simulink model "Separately_excited_DC_motor"  (R2024a)
settings: Solver=ode15s  StartTime=0.0  StopTime=35  RelTol=1e-3
values from neighbouring files (symbols this model uses):
  A = 1.4    [CruiseControl.m]
libraries: slpidlib x2, spsControlledVoltageSourceLib x2, spsGroundLib x2, spsDCMachineLib x1, SignalEditorBlockLib x1, sps_lib x1
settings Model: Creator=macbookair  LastModifiedBy=macbookair

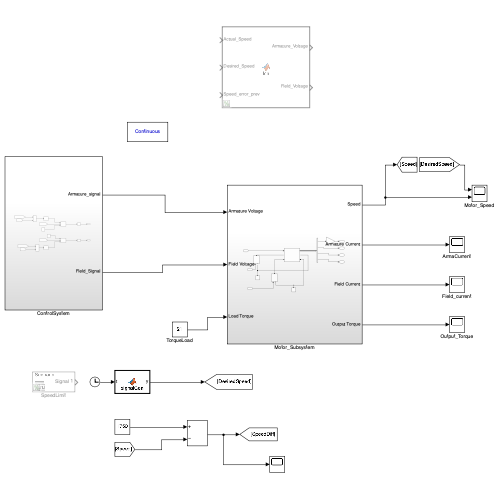
[thumbnail: Simulink's stored preview of the top-level diagram]
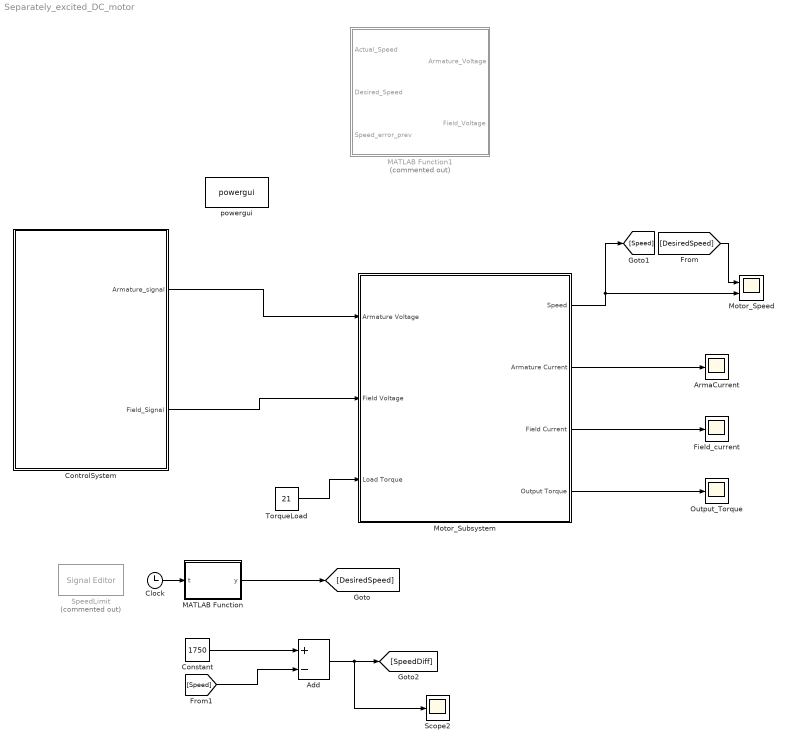
== system Separately_excited_DC_motor ==
  Add : Sum  Inputs=+-
  ArmaCurrent : Scope
  Clock : Clock
  Constant : Constant  Value=1750
  ControlSystem : Subsystem
  Field_current : Scope
  MATLAB Function : MATLAB Function  TreatAsAtomicUnit=on
  MATLAB Function1 : MATLAB Function  Commented=on  TreatAsAtomicUnit=on
  Motor_Speed : Scope  NumInputPorts=2
  Motor_Subsystem : Subsystem
  Output_Torque : Scope
  Scope2 : Scope
  SpeedLimit : SignalEditorBlockLib/Signal Editor  Commented=on  FileName=SpeedLimit.mat  ActiveScenario=Scenario  ActiveSignal=Signal 1  IsBus=off  OutputBusObjectStr=Bus: BusObject  SampleTime=0  Interpolate=off  ZeroCross=off  OutputAfterFinalValue=Setting to zero  Unit=inherit  PreserveSignalName=on  ApplySigPropsToAllScenarios=on  ApplySigPropsToAllSignals=off
  TorqueLoad : Constant  Value=21
  powergui : sps_lib/powergui  Priority=1  SimulationMode=Continuous  SampleTime=50e-6  frequency=60  Iterations=50  frequencyindice=0  Pbase=100e6  ErrMax=1e-4  UnitsV=kV  UnitsW=MW  buscounter=0  FunctionMessages=off  echomessages=off  EnableUseOfTLC=off  CurrentSourceSwitches=off  DisableSnubberDevices=off  DisableRonSwitches=off  DisableVfSwitches=off  DisplayEquations=off  AutomaticDiscreteSolvers=off  SolverType=Tustin/Backward Euler (TBE)  Interpol=off  ExternalGateDelay=off  methode=off  Ts=100  x0status=blocks  SPID=on  SwTol=0  HookPort=off  NonlinearTolerance=1e-4  nMaxIteration=100  ContinueOnMaxIteration=off  RestoreLinks=warning  ResistiveCurrentMeasurement=off  Frange=[0:2:500]  Ylog=off  Xlog=on  ShowGrid=off  save=off  variable=ZData  structure=0  ZoomFFT=off  StartTime=0.0  cycles=1  DisplayStyle=1  fundamental=60  FreqAxis=off  MaxFrequency=1000  frequencyindicesteady=1  RmsSteady=1  display=off
  wires:
  Motor_Subsystem/2(Armature Current) -> ArmaCurrent/1
  Motor_Subsystem/4(Output Torque) -> Output_Torque/1
  Motor_Subsystem/3(Field Current) -> Field_current/1
  Motor_Subsystem/1(Speed) -> Motor_Speed/2, [Speed]
  [DesiredSpeed] -> Motor_Speed/1
  [Speed] -> Add/2
  Constant/1 -> Add/1
  Add/1 -> Scope2/1, [SpeedDiff]
  TorqueLoad/1 -> Motor_Subsystem/3(Load Torque)
  Clock/1 -> MATLAB Function/1(t)
  MATLAB Function/1(y) -> [DesiredSpeed]
  ControlSystem/1(Armature_signal) -> Motor_Subsystem/1(Armature Voltage)
  ControlSystem/2(Field_Signal) -> Motor_Subsystem/2(Field Voltage)

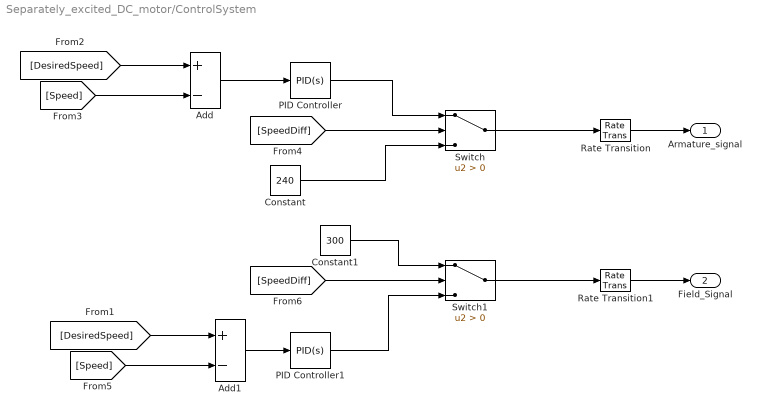
== system Separately_excited_DC_motor/ControlSystem ==
  Add : Sum  Inputs=+-
  Add1 : Sum  Inputs=+-
  Constant : Constant  Value=240
  Constant1 : Constant  Value=300
  PID Controller : slpidlib/PID Controller  Controller=PID  Form=Parallel  TimeDomain=Continuous-time  UseExternalTs=off  SampleTime=-1  IntegratorMethod=Forward Euler  FilterMethod=Forward Euler  ControllerParametersSource=internal  P=100  I=50  UseKiTs=off  D=0.001  UseExternalDerivativeSource=off  N=100  UseFilter=on  TunerSelectOption=Transfer Function Based (PID Tuner App)  InitialConditionSource=internal  InitialConditionForIntegrator=0  InitialConditionForFilter=0  DifferentiatorICPrevScaledInput=0  ExternalReset=none  TrackingMode=off  Kt=1  LimitOutput=off  SatLimitsSource=internal  UpperSaturationLimit=inf  LowerSaturationLimit=-inf  LinearizeAsGain=on  AntiWindupMode=none  Kb=1  LimitIntegrator=off  UpperIntegratorSaturationLimit=inf  LowerIntegratorSaturationLimit=-inf  POutMin=[]  POutMax=[]  IOutMin=[]  IOutMax=[]  DOutMin=[]  DOutMax=[]  NOutMin=[]  NOutMax=[]  SumOutMin=[]  SumOutMax=[]  SaturationOutMin=[]  SaturationOutMax=[]  PParamMin=[]  PParamMax=[]  IParamMin=[]  IParamMax=[]  DParamMin=[]  DParamMax=[]  NParamMin=[]  NParamMax=[]  KbParamMin=[]  KbParamMax=[]  KtParamMin=[]  KtParamMax=[]  KbOutMin=[]  KbOutMax=[]  KtOutMin=[]  KtOutMax=[]  IntegratorOutMin=[]  IntegratorOutMax=[]  FilterOutMin=[]  FilterOutMax=[]  SumI1OutMin=[]  SumI1OutMax=[]  SumI2OutMin=[]  SumI2OutMax=[]  SumI3OutMin=[]  SumI3OutMax=[]  SumI4OutMin=[]  SumI4OutMax=[]  SumDOutMin=[]  SumDOutMax=[]  DifferentiatorOutMin=[]  DifferentiatorOutMax=[]  FilterDiffOutCoefMin=[]  FilterDiffOutCoefMax=[]  ReciprocalOutMin=[]  ReciprocalOutMax=[]  SumDenOutMin=[]  SumDenOutMax=[]  SumNumOutMin=[]  SumNumOutMax=[]  DivideOutMin=[]  DivideOutMax=[]  UdiffTsProdOutMin=[]  UdiffTsProdOutMax=[]  NTsProdOutMin=[]  NTsProdOutMax=[]  UintegralTsProdOutMin=[]  UintegralTsProdOutMax=[]  UngainTsProdOutMin=[]  UngainTsProdOutMax=[]  ClampingZeroOutDataTypeStr=Inherit: Inherit via back propagation  ClampingZeroOutMin=[]  ClampingZeroOutMax=[]  FilterDenConstantOutDataTypeStr=Inherit: Inherit via back propagation  FilterDenConstantOutMin=[]  FilterDenConstantOutMax=[]  PCopyOutDataTypeStr=Inherit: Inherit via back propagation  PCopyOutMin=[]  PCopyOutMax=[]  NCopyOutDataTypeStr=Inherit: Inherit via back propagation  NCopyOutMin=[]  NCopyOutMax=[]  IntegratorContinuousStateAttributes=''  IntegratorStateMustResolveToSignalObject=off  IntegratorRTWStateStorageClass=Auto  FilterContinuousStateAttributes=''  FilterStateMustResolveToSignalObject=off  FilterRTWStateStorageClass=Auto  ParallelPVariant=InternalParameters  IdealPVariant=Disabled  IVariant=InternalParameters  DVariant=InternalParameters  IntegratorVariant=Continuous  SatVariant=Disabled  AWVariant=Passthrough  PCopyVariant=Disabled  TRVariant=Disabled  FdbkBlocksVariant=Forward  IdealPFdbkVariant=Disabled  SatFdbkVariant=Disabled  DerivativeFilterVariant=ContFilter  NVariant=InternalParameters  NCopyVariant=Disabled  FilterICVariant=InternalICsFilter  IntegratorICVariant=InternalICs  ExternalResetVariant=Disabled  TRSumVariant=Passthrough  SumFdbkVariant=Disabled  SumVariant=Sum_PID  TsampFilterVariant=InternalTs  TsampNgainVariant=Passthrough  TsampIntegralVariant=Disabled_SignalSpec  ExternalSaturationOutDataTypeStr=Inherit: Same as second input  DerivativeSourceVariant=ErrorSignal
  PID Controller1 : slpidlib/PID Controller  Controller=PID  Form=Parallel  TimeDomain=Continuous-time  UseExternalTs=off  SampleTime=-1  IntegratorMethod=Forward Euler  FilterMethod=Forward Euler  ControllerParametersSource=internal  P=200  I=40  UseKiTs=off  D=0.001  UseExternalDerivativeSource=off  N=100  UseFilter=on  TunerSelectOption=Transfer Function Based (PID Tuner App)  InitialConditionSource=internal  InitialConditionForIntegrator=0  InitialConditionForFilter=0  DifferentiatorICPrevScaledInput=0  ExternalReset=none  TrackingMode=off  Kt=1  LimitOutput=off  SatLimitsSource=internal  UpperSaturationLimit=inf  LowerSaturationLimit=-inf  LinearizeAsGain=on  AntiWindupMode=none  Kb=1  LimitIntegrator=off  UpperIntegratorSaturationLimit=inf  LowerIntegratorSaturationLimit=-inf  POutMin=[]  POutMax=[]  IOutMin=[]  IOutMax=[]  DOutMin=[]  DOutMax=[]  NOutMin=[]  NOutMax=[]  SumOutMin=[]  SumOutMax=[]  SaturationOutMin=[]  SaturationOutMax=[]  PParamMin=[]  PParamMax=[]  IParamMin=[]  IParamMax=[]  DParamMin=[]  DParamMax=[]  NParamMin=[]  NParamMax=[]  KbParamMin=[]  KbParamMax=[]  KtParamMin=[]  KtParamMax=[]  KbOutMin=[]  KbOutMax=[]  KtOutMin=[]  KtOutMax=[]  IntegratorOutMin=[]  IntegratorOutMax=[]  FilterOutMin=[]  FilterOutMax=[]  SumI1OutMin=[]  SumI1OutMax=[]  SumI2OutMin=[]  SumI2OutMax=[]  SumI3OutMin=[]  SumI3OutMax=[]  SumI4OutMin=[]  SumI4OutMax=[]  SumDOutMin=[]  SumDOutMax=[]  DifferentiatorOutMin=[]  DifferentiatorOutMax=[]  FilterDiffOutCoefMin=[]  FilterDiffOutCoefMax=[]  ReciprocalOutMin=[]  ReciprocalOutMax=[]  SumDenOutMin=[]  SumDenOutMax=[]  SumNumOutMin=[]  SumNumOutMax=[]  DivideOutMin=[]  DivideOutMax=[]  UdiffTsProdOutMin=[]  UdiffTsProdOutMax=[]  NTsProdOutMin=[]  NTsProdOutMax=[]  UintegralTsProdOutMin=[]  UintegralTsProdOutMax=[]  UngainTsProdOutMin=[]  UngainTsProdOutMax=[]  ClampingZeroOutDataTypeStr=Inherit: Inherit via back propagation  ClampingZeroOutMin=[]  ClampingZeroOutMax=[]  FilterDenConstantOutDataTypeStr=Inherit: Inherit via back propagation  FilterDenConstantOutMin=[]  FilterDenConstantOutMax=[]  PCopyOutDataTypeStr=Inherit: Inherit via back propagation  PCopyOutMin=[]  PCopyOutMax=[]  NCopyOutDataTypeStr=Inherit: Inherit via back propagation  NCopyOutMin=[]  NCopyOutMax=[]  IntegratorContinuousStateAttributes=''  IntegratorStateMustResolveToSignalObject=off  IntegratorRTWStateStorageClass=Auto  FilterContinuousStateAttributes=''  FilterStateMustResolveToSignalObject=off  FilterRTWStateStorageClass=Auto  ParallelPVariant=InternalParameters  IdealPVariant=Disabled  IVariant=InternalParameters  DVariant=InternalParameters  IntegratorVariant=Continuous  SatVariant=Disabled  AWVariant=Passthrough  PCopyVariant=Disabled  TRVariant=Disabled  FdbkBlocksVariant=Forward  IdealPFdbkVariant=Disabled  SatFdbkVariant=Disabled  DerivativeFilterVariant=ContFilter  NVariant=InternalParameters  NCopyVariant=Disabled  FilterICVariant=InternalICsFilter  IntegratorICVariant=InternalICs  ExternalResetVariant=Disabled  TRSumVariant=Passthrough  SumFdbkVariant=Disabled  SumVariant=Sum_PID  TsampFilterVariant=InternalTs  TsampNgainVariant=Passthrough  TsampIntegralVariant=Disabled_SignalSpec  ExternalSaturationOutDataTypeStr=Inherit: Same as second input  DerivativeSourceVariant=ErrorSignal
  Rate Transition : RateTransition
  Rate Transition1 : RateTransition
  Switch : Switch  Criteria=u2 > Threshold  SaturateOnIntegerOverflow=off  InputSameDT=off
  Switch1 : Switch  Criteria=u2 > Threshold  SaturateOnIntegerOverflow=off  InputSameDT=off
  Armature_signal : Outport
  Field_Signal : Outport  Port=2
  wires:
  Add/1 -> PID Controller/1
  Add1/1 -> PID Controller1/1
  [Speed] -> Add/2
  [DesiredSpeed] -> Add/1
  [DesiredSpeed] -> Add1/1
  [Speed] -> Add1/2
  [SpeedDiff] -> Switch/2
  [SpeedDiff] -> Switch1/2
  PID Controller1/1 -> Switch1/3
  Constant/1 -> Switch/3
  Constant1/1 -> Switch1/1
  PID Controller/1 -> Switch/1
  Switch1/1 -> Rate Transition1/1
  Switch/1 -> Rate Transition/1
  Rate Transition1/1 -> Field_Signal/1
  Rate Transition/1 -> Armature_signal/1

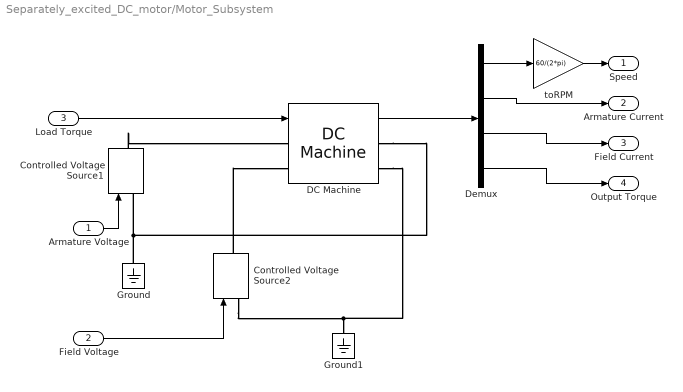
== system Separately_excited_DC_motor/Motor_Subsystem ==
  Armature Voltage : Inport
  Field Voltage : Inport  Port=2
  Load Torque : Inport  Port=3
  Controlled Voltage Source1 : spsControlledVoltageSourceLib/Controlled Voltage Source  Initialize=on  Source_Type=AC  Amplitude=0  Phase=0  Frequency=0  Measurements=None
  Controlled Voltage Source2 : spsControlledVoltageSourceLib/Controlled Voltage Source  Initialize=on  Source_Type=AC  Amplitude=0  Phase=0  Frequency=0  Measurements=None
  DC Machine : spsDCMachineLib/DC Machine  PresetModel=01: 5HP 240V 1750RPM Field:300V  MechanicalLoad=Torque TL  FieldType=Wound  ShowDetailedParameters=on  MeasurementBus=off  RLa=[2.581 0.028]  RLf=[281.2 156]  Laf=0.9483  MachineConstant=Torque constant (N.m/A)  Ke=1.8  Kt=1.8  J=0.02215  Bm=0.002953  Tf=0.5161  w0=1  Ifinit=0  TsPowergui=0  TsBlock=-1
  Demux : Demux
  Ground : spsGroundLib/Ground  LConnTagsString=a
  Ground1 : spsGroundLib/Ground  LConnTagsString=a
  toRPM : Gain  Gain=60/(2*pi)
  Speed : Outport
  Armature Current : Outport  Port=2
  Field Current : Outport  Port=3
  Output Torque : Outport  Port=4
  wires:
  Field Voltage/1 -> Controlled Voltage Source2/1
  Demux/2 -> Armature Current/1
  Demux/4 -> Output Torque/1
  Demux/3 -> Field Current/1
  Armature Voltage/1 -> Controlled Voltage Source1/1
  Demux/1 -> toRPM/1
  DC Machine/1 -> Demux/1
  toRPM/1 -> Speed/1
  Load Torque/1 -> DC Machine/1
  connections:
  Controlled Voltage Source1/RConn1 -- DC Machine/LConn1
  Ground/LConn1 -- DC Machine/RConn1 -- Controlled Voltage Source1/LConn1
  Controlled Voltage Source2/RConn1 -- DC Machine/LConn2
  Controlled Voltage Source2/LConn1 -- DC Machine/RConn2 -- Ground1/LConn1

== matlab function Separately_excited_DC_motor/MATLAB Function1 ==
  data: Actual_Speed input; Armature_Voltage output; Desired_Speed input; Field_Voltage output; Speed_error_prev input
function [Armature_Voltage, Field_Voltage] = fcn(Actual_Speed, Desired_Speed, Speed_error_prev)

    Rated_Speed = 1750; % rpm
    Rated_Armature_Voltage = 240; 
    Rated_Field_Voltage = 300; 
  
    Speed_difference = Rated_Speed - Actual_Speed;
    Speed_error = Actual_Speed - Desired_Speed;
    
    Kp = 0.1;  
    Ki = 0.01; 
    Kd = 0.001; 
    
   
    PID_output = Kp * Speed_error ; 
    
    if Speed_difference > 0
        % Armature Control Mode (Speed < 1750 rpm)
        Armature_Voltage = Rated_Armature_Voltage + PID_output;
        Field_Voltage = Rated_Field_Voltage;
    else
        % Field Weakening Mode (Speed >= 1750 rpm)
        Armature_Voltage = Rated_Armature_Voltage;
        Field_Voltage = Rated_Field_Voltage - PID_output;
    end
    
    % Limit outputs to reasonable ranges
    Armature_Voltage = min(max(Armature_Voltage, 0), 300);
    Field_Voltage = min(max(Field_Voltage, 0), 300);
end

== matlab function Separately_excited_DC_motor/MATLAB Function ==
  data: t input; y output
function y = signalGen(t)
% Custom signal generator

if t < 0
    y = 0;
elseif t >= 0 && t < 15
    y = (2000 / 15) * t;
elseif t >= 15 && t < 20
    y = 2000;
elseif t >= 20 && t <= 35
    y = 2000 - ((2000 / 15) * (t - 20));
else
    y = 0;
end
